simulink model "filtro_ECG1"  (R2019b)
settings: Solver=VariableStepAuto  StartTime=0.0  StopTime=1  RelTol=1e-3
values from neighbouring files (symbols this model uses):
  T = 0.00833333333333    [ECG_graficos_fft.mat]    (also in FPB_Arduino.mat = 0.001; butter1.mat = 1.25e-08; filtro_notch1.mat; intro_resp_freq.mat = 0.00125)
settings Model: Creator=fernandopassold  LastModifiedBy=fernandopassold

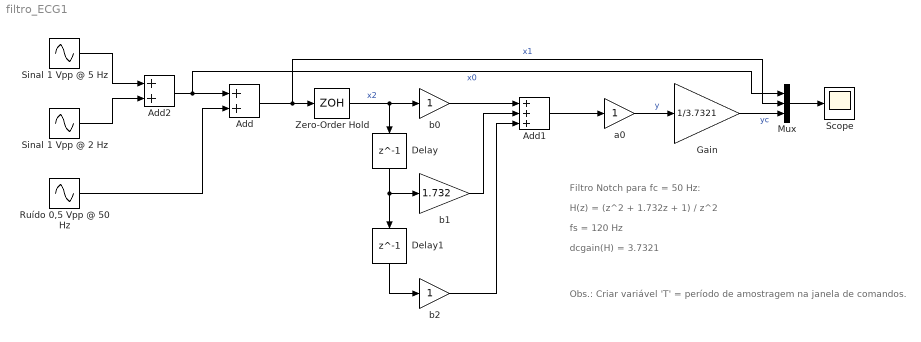
== system filtro_ECG1 ==
  note: dcgain(H) = 3.7321
  note: fs = 120 Hz
  note: Filtro Notch para fc = 50 Hz:
  note: H(z) = (z^2 + 1.732z + 1) / z^2
  note: Obs.: Criar variável 'T' = período de amostragem na janela de comandos.
  Add : Sum
  Add1 : Sum  Inputs=+++
  Add2 : Sum
  Delay : Delay  DelayLength=1  SampleTime=T
  Delay1 : Delay  DelayLength=1  SampleTime=T
  Gain : Gain  Gain=1/3.7321
  Mux : Mux  Inputs=3
  Ruído 0,5 Vpp @ 50 Hz : Sin  Amplitude=0.5  Frequency=2*pi*50  Phase=pi/2  SampleTime=1/500
  Scope : Scope
  Sinal 1 Vpp @ 2 Hz : Sin  Frequency=2*pi*2  Phase=pi/2  SampleTime=1/200
  Sinal 1 Vpp @ 5 Hz : Sin  Frequency=2*pi*5  SampleTime=1/50
  "Zero-Order Hold " : ZeroOrderHold  SampleTime=T
  a0 : Gain
  b0 : Gain
  b1 : Gain  Gain=1.732
  b2 : Gain
  wires:
  b0/1 -> Add1/1
  Delay/1 -> Delay1/1, b1/1
  b1/1 -> Add1/2
  Delay1/1 -> b2/1
  b2/1 -> Add1/3
  Mux/1 -> Scope/1
  Add/1 -> Mux/2, "Zero-Order Hold "/1  "x1"
  "Zero-Order Hold "/1 -> Delay/1, b0/1  "x2"
  Add2/1 -> Mux/1, Add/1  "x0"
  Sinal 1 Vpp @ 5 Hz/1 -> Add2/1
  Sinal 1 Vpp @ 2 Hz/1 -> Add2/2
  Ruído 0,5 Vpp @ 50 Hz/1 -> Add/2
  a0/1 -> Gain/1  "y"
  Gain/1 -> Mux/3  "yc"
  Add1/1 -> a0/1
